simulink model "symuEj10"  (R2021a)
settings: Solver=VariableStepAuto  StartTime=0.0  StopTime=20  RelTol=1e-3
InitFcn:
  | symuej10
undefined symbols (not defined in the file): b, d1, d2, f1, k, m
settings Model: Creator=LabF103_PC12  LastModifiedBy=LabF103_PC12

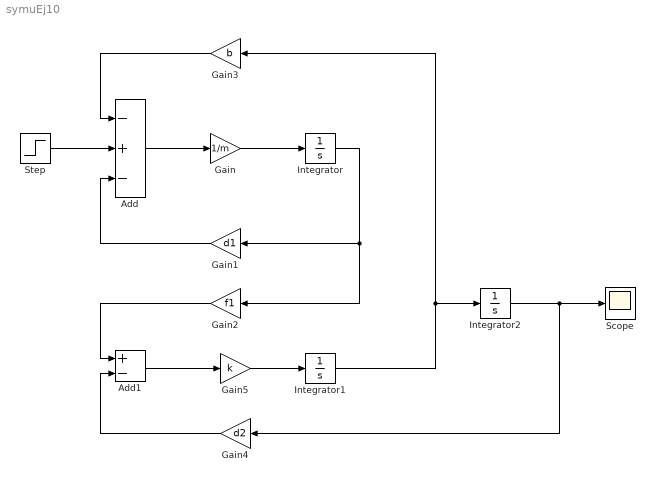
== system symuEj10 ==
  Add : Sum  Inputs=-+-
  Add1 : Sum  Inputs=+-
  Gain : Gain  Gain=1/m
  Gain1 : Gain  Gain=d1
  Gain2 : Gain  Gain=f1
  Gain3 : Gain  Gain=b
  Gain4 : Gain  Gain=d2
  Gain5 : Gain  Gain=k
  Integrator : Integrator
  Integrator1 : Integrator
  Integrator2 : Integrator
  Scope : Scope
  Step : Step  Time=0  SampleTime=0
  wires:
  Step/1 -> Add/2
  Add/1 -> Gain/1
  Gain3/1 -> Add/1
  Gain/1 -> Integrator/1
  Integrator/1 -> Gain2/1, Gain1/1
  Gain1/1 -> Add/3
  Gain2/1 -> Add1/1
  Gain4/1 -> Add1/2
  Add1/1 -> Gain5/1
  Gain5/1 -> Integrator1/1
  Integrator2/1 -> Gain4/1, Scope/1
  Integrator1/1 -> Integrator2/1, Gain3/1
